simulink model "Test_Word_Multiplexer_4_to_1_DirSel"  (Simulink 8.7)
settings: Solver=ode45  StartTime=0.0  StopTime=len  RelTol=1e-3
libraries: Miscellaneous x5, commutil2 x1, Word_Multiplexers_Lib x1
settings Model: Creator=N  LastModifiedBy=Jozko Mrkvicka
settings DataIOCC: LimitDataPoints=off
settings DebuggingCC: UnderspecifiedInitializationDetection=Simplified  MergeDetectMultiDrivingBlocksExec=error
settings HardwareCC: ProdBitPerPointer=64  ProdLargestAtomicFloat=Float  ProdIntDivRoundTo=Zero  ProdEndianess=LittleEndian  ProdHWDeviceType=Intel->x86-64 (Windows64)
settings ModelReferenceCC: PropagateSignalLabelsOutOfModel=on

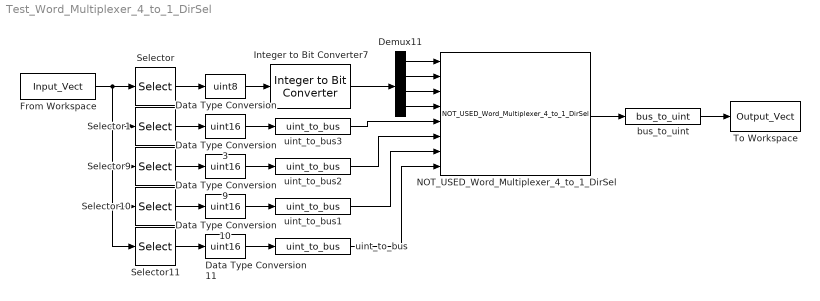
== system Test_Word_Multiplexer_4_to_1_DirSel ==
  Data Type Conversion : DataTypeConversion  OutDataTypeStr=uint8
  Data Type Conversion{3,9..11} (4 alike) : DataTypeConversion  OutDataTypeStr=uint16
  Demux11 : Demux
  From Workspace : FromWorkspace  VariableName=Input_Vect  SampleTime=1  Interpolate=off  OutputAfterFinalValue=Holding final value
  Integer to Bit Converter7 : commutil2/Integer to Bit Converter  nbits=4  signedInputValues=Unsigned  bitOrder=MSB first  outDtype=boolean
  NOT_USED_Word_Multiplexer_4_to_1_DirSel : Word_Multiplexers_Lib/Word_Multiplexers_Lib/NOT_USED_Word_Multiplexer_4_to_1_DirSel
  Selector : Selector  IndexMode=Zero-based  InputPortWidth=5  SampleTime=1  IndexOptions=Index vector (dialog)  Indices=0  OutputSizes=1
  Selector1 : Selector  IndexMode=Zero-based  InputPortWidth=5  IndexOptions=Index vector (dialog)  Indices=1  OutputSizes=1
  Selector10 : Selector  IndexMode=Zero-based  InputPortWidth=5  IndexOptions=Index vector (dialog)  Indices=3  OutputSizes=1
  Selector11 : Selector  IndexMode=Zero-based  InputPortWidth=5  IndexOptions=Index vector (dialog)  Indices=4  OutputSizes=1
  Selector9 : Selector  IndexMode=Zero-based  InputPortWidth=5  IndexOptions=Index vector (dialog)  Indices=2  OutputSizes=1
  To Workspace : ToWorkspace  VariableName=Output_Vect  SampleTime=1
  bus_to_uint : Miscellaneous/bus_to_uint
  uint_to_bus{,1..3} (4 alike) : Miscellaneous/uint_to_bus
  wires:
  NOT_USED_Word_Multiplexer_4_to_1_DirSel/1 -> bus_to_uint/1
  Integer to Bit Converter7/1 -> Demux11/1
  Selector/1 -> Data Type Conversion/1
  Selector1/1 -> Data Type Conversion3/1
  Data Type Conversion3/1 -> uint_to_bus3/1
  Data Type Conversion/1 -> Integer to Bit Converter7/1
  Selector9/1 -> Data Type Conversion9/1
  From Workspace/1 -> Selector11/1, Selector10/1, Selector9/1, Selector1/1, Selector/1
  Selector10/1 -> Data Type Conversion10/1
  Selector11/1 -> Data Type Conversion11/1
  Data Type Conversion9/1 -> uint_to_bus2/1
  Data Type Conversion10/1 -> uint_to_bus1/1
  Data Type Conversion11/1 -> uint_to_bus/1
  uint_to_bus3/1 -> NOT_USED_Word_Multiplexer_4_to_1_DirSel/5
  uint_to_bus2/1 -> NOT_USED_Word_Multiplexer_4_to_1_DirSel/6
  uint_to_bus1/1 -> NOT_USED_Word_Multiplexer_4_to_1_DirSel/7
  uint_to_bus/1 -> NOT_USED_Word_Multiplexer_4_to_1_DirSel/8
  bus_to_uint/1 -> To Workspace/1
  Demux11/1 -> NOT_USED_Word_Multiplexer_4_to_1_DirSel/1
  Demux11/2 -> NOT_USED_Word_Multiplexer_4_to_1_DirSel/2
  Demux11/3 -> NOT_USED_Word_Multiplexer_4_to_1_DirSel/3
  Demux11/4 -> NOT_USED_Word_Multiplexer_4_to_1_DirSel/4
